simulink model "lab4_blinkLed"  (R2015a)
settings: Solver=ode45  StartTime=0.0  StopTime=10.0  RelTol=1e-3
settings Model: Creator=mt  LastModifiedBy=blds3

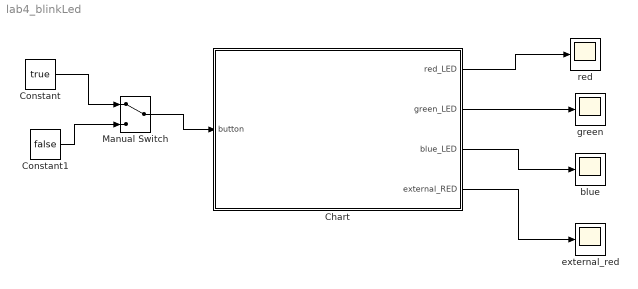
== system lab4_blinkLed ==
  Chart : Stateflow chart  TreatAsAtomicUnit=on
  Constant : Constant  Value=true
  Constant1 : Constant  Value=false
  Manual Switch : ManualSwitch
  blue : Scope
      settings: SaveName=ScopeData2
  external_red : Scope
      settings: SaveName=ScopeData3
  green : Scope
  red : Scope
  wires:
  Constant/1 -> Manual Switch/1
  Constant1/1 -> Manual Switch/2
  Manual Switch/1 -> Chart/1(button)
  Chart/1(red_LED) -> red/1
  Chart/2(green_LED) -> green/1
  Chart/3(blue_LED) -> blue/1
  Chart/4(external_RED) -> external_red/1

== stateflow chart lab4_blinkLed/Chart ==
  state LedOff
    entry: external_RED=false;
    red_LED=false;
    green_LED=false;
    blue_LED=false
  state LedOn
    entry: external_RED=true;
    red_LED=true;
    green_LED=true;
    blue_LED=true
  (junction 27) -> LedOff [order 2]
  (default) -> LedOff
  (junction 9) -> LedOn [order 2]
  LedOff -> (junction 9) : {i=0}
  LedOn -> (junction 27) : {i=0}
  (junction 9) -> (junction 10) [order 1] : [i<10]
  (junction 27) -> (junction 22) [order 1] : [i<10]
  (junction 10) -> (junction 9) : {i = i + 1}
  (junction 22) -> (junction 27) : {i = i + 1}
  data: button input boolean; red_LED output boolean; green_LED output boolean; blue_LED output boolean; external_RED output boolean; i local
